simulink model "Galvo_sys_v1mmm3"  (R2013a)
settings: Solver=ode45  StartTime=0.0  StopTime=30e-3  MaxStep=1e-5  RelTol=1e-3
PreLoadFcn:
  | %Tfin = get_param(gcs,'Tfin');
  | %Kp_cc = evalin('base',paramCtrl.Kp_cc);
  | %CC_EN = 1;
  | %Kp_ccMod = Kp_cc;
model workspace (MATLAB code in the model file):
  | set_param(gcs,'Tfin',num2str(evalin('base', 'Tfin')));
  | Tfin=str2num(get_param(gcs,'Tfin'));
  | CC_EN = 1
  | Kp3=1
undefined symbols (not defined in the file or in its folder): Kp_cc
libraries: simulink x2
settings Model: CC_EN=1  Tfin=0.01  TunableVars=Kp3  TunableVarsStorageClass=Auto  BufferReuse=off  Creator=mainster  LastModifiedBy=mainster
settings DataIOCC: LimitDataPoints=off  SaveOutput=off  SignalLogging=off  DSMLogging=off  SaveTime=off
settings OptimizationCC: BlockReduction=off  InlineParams=on  InlineInvariantSignals=on  OptimizeBlockIOStorage=off  BufferReuse=off  ExpressionFolding=off  LocalBlockOutputs=off
settings DebuggingCC: InitInArrayFormatMsg=none

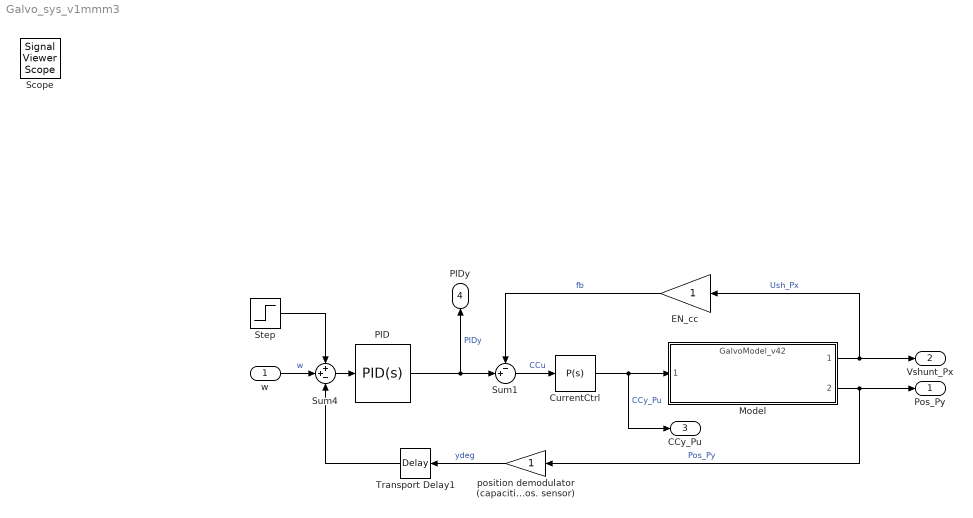
== system Galvo_sys_v1mmm3 ==
  w : Inport
  CurrentCtrl : simulink/Continuous/PID Controller  Controller=P  TimeDomain=Continuous-time  SampleTime=1  IntegratorMethod=Forward Euler  FilterMethod=Forward Euler  Form=Parallel  P=Kp_cc  I=1  D=0  N=100  InitialConditionSource=internal  InitialConditionForIntegrator=0  InitialConditionForFilter=0  ExternalReset=none  LimitOutput=on  UpperSaturationLimit=25  LowerSaturationLimit=-25  LinearizeAsGain=on  AntiWindupMode=none  Kb=1  TrackingMode=off  Kt=1  PParamMin=[]  PParamMax=[]  IParamMin=[]  IParamMax=[]  DParamMin=[]  DParamMax=[]  NParamMin=[]  NParamMax=[]  KbParamMin=[]  KbParamMax=[]  KtParamMin=[]  KtParamMax=[]  POutMin=[]  POutMax=[]  IOutMin=[]  IOutMax=[]  DOutMin=[]  DOutMax=[]  NOutMin=[]  NOutMax=[]  KbOutMin=[]  KbOutMax=[]  KtOutMin=[]  KtOutMax=[]  IntegratorOutMin=[]  IntegratorOutMax=[]  FilterOutMin=[]  FilterOutMax=[]  SumOutMin=[]  SumOutMax=[]  SumI1OutMin=[]  SumI1OutMax=[]  SumI2OutMin=[]  SumI2OutMax=[]  SumI3OutMin=[]  SumI3OutMax=[]  SumDOutMin=[]  SumDOutMax=[]  SaturationOutMin=[]  SaturationOutMax=[]  IntegratorContinuousStateAttributes=''  IntegratorStateMustResolveToSignalObject=off  IntegratorRTWStateStorageClass=Auto  FilterContinuousStateAttributes=''  FilterStateMustResolveToSignalObject=off  FilterRTWStateStorageClass=Auto
      settings: AttributesFormatString=Kp_cc = %<P>\nUccLim = +-%<UpperSaturationLimit>
  EN_cc : Gain
  Model : ModelReference  ModelNameDialog=GalvoModel_v42.slx  SimulationMode=Normal  ModelReferenceVersion=1.13  CopyOfModelName=GalvoModel_v42.slx  DefaultDataLogging=on
      mask Display:
      | str=sprintf('%s',get(gcbh,'ModelName'));
      | port_label('input', 1, 'VCoil','texmode','on')
      | color('blue');
      | port_label('output', 1, 'VShunt','texmode','on')
      | color('black');
      | port_label('output', 2, 'AngPos')
      | %text(.05,.98,['{\fontsize{12}\it\bf' strrep(str,'_',' ') '}'],'horizontalAlignment','left','verticalAlignment','top','texmode','on')
      | text(.015,.98,['{\fontsize{12}\it\bf' strrep(str,'_','\_') '}'],'horizontalAlignment','left','verticalAlignment','top','texmode','on')
  PID : simulink/Continuous/PID Controller  Controller=PID  TimeDomain=Continuous-time  SampleTime=1  IntegratorMethod=Forward Euler  FilterMethod=Forward Euler  Form=Ideal  P=1.14533423709275  I=9.52023676976267  D=0.0126974512595782  N=3428.84832659657  InitialConditionSource=internal  InitialConditionForIntegrator=0  InitialConditionForFilter=0  ExternalReset=none  IgnoreLimit=on  LimitOutput=on  UpperSaturationLimit=2.5  LowerSaturationLimit=-2.5  LinearizeAsGain=on  AntiWindupMode=back-calculation  Kb=6  TrackingMode=off  Kt=0  PParamMin=[]  PParamMax=[]  IParamMin=[]  IParamMax=[]  DParamMin=[]  DParamMax=[]  NParamMin=[]  NParamMax=[]  KbParamMin=[]  KbParamMax=[]  KtParamMin=[]  KtParamMax=[]  POutMin=[]  POutMax=[]  IOutMin=[]  IOutMax=[]  DOutMin=[]  DOutMax=[]  NOutMin=[]  NOutMax=[]  KbOutMin=[]  KbOutMax=[]  KtOutMin=[]  KtOutMax=[]  IntegratorOutMin=[]  IntegratorOutMax=[]  FilterOutMin=[]  FilterOutMax=[]  SumOutMin=[]  SumOutMax=[]  SumI1OutMin=[]  SumI1OutMax=[]  SumI2OutMin=[]  SumI2OutMax=[]  SumI3OutMin=[]  SumI3OutMax=[]  SumDOutMin=[]  SumDOutMax=[]  SaturationOutMin=[]  SaturationOutMax=[]  IntegratorContinuousStateAttributes=''  IntegratorStateMustResolveToSignalObject=off  IntegratorRTWStateStorageClass=Auto  FilterContinuousStateAttributes=''  FilterStateMustResolveToSignalObject=off  FilterRTWStateStorageClass=Auto
      settings: AttributesFormatString=AWM=%<AntiWindupMode>\nD=%<D>\nI=%<I>\nN=%<N>\nP=%<P>\nLimit=+-%<UpperSaturationLimit>
  Step : Step  Time=1e-3  SampleTime=0  ZeroCross=off
      settings: AttributesFormatString=Ampl.: %<After>
  Sum1 : Sum  Inputs=-+|
  Sum4 : Sum  Inputs=++-
  Transport Delay1 : TransportDelay  DelayTime=1e-6
  position demodulator (capacitive angular pos. sensor) : Gain
  Pos_Py : Outport
  Vshunt_Px : Outport  Port=2
  CCy_Pu : Outport  Port=3
  PIDy : Outport  Port=4
  Scope : SignalViewerScope  IOType=viewer  NumInputPorts=4  RefreshTime=0.035000
      settings: ShowLegends=on  TimeRange=0.03  YMin=-0.2~-2~-2~-0.1  YMax=1~3~3~0.15  MaxDataPoints=75000
  wires:
  Sum4/1 -> PID/1
  Step/1 -> Sum4/1
  w/1 -> Sum4/2  "w"
  position demodulator (capacitive angular pos. sensor)/1 -> Transport Delay1/1  "ydeg"
  Model/1 -> Vshunt_Px/1, EN_cc/1  "Ush_Px"
  Sum1/1 -> CurrentCtrl/1  "CCu"
  PID/1 -> Sum1/2, PIDy/1  "PIDy"
  Model/2 -> Pos_Py/1, position demodulator (capacitive angular pos. sensor)/1  "Pos_Py"
  EN_cc/1 -> Sum1/1  "fb"
  Transport Delay1/1 -> Sum4/3
  CurrentCtrl/1 -> Model/1, CCy_Pu/1  "CCy_Pu"
